simulink model "XianKongTest2022b"  (R2021a)
settings: Solver=VariableStepAuto  StartTime=0.0  StopTime=10.0  RelTol=1e-3
values from neighbouring files (symbols this model uses):
  A = [ 0 0 1 0 ... (first row only)    [fang_daolibai.m]    (also in xiankongdlb.m = [     0       0         1         0)
  B = [0;0;5.2184;-6.5125]    [fang_daolibai.m]    (also in xiankongdlb.m)
  C = [1,0,0,0;0,1,0,0]    [fang_daolibai.m]    (also in xiankongdlb.m)
  K = [  -60.6992 -316.1745  -30.0745  -33.7643]    [daolibai.m]    (also in dlfun.m = [ -60.6992 -316.1745  -30.0745  -33.7643]; fang_daolibai.m = place(A,B,P); xiankongdlb.m = place(A,B,P))
  L = place(A',C',P1)'    [fang_daolibai.m]    (also in xiankongdlb.m)
settings Model: Creator=DELL  LastModifiedBy=HanDong
settings SolverCC: AlgebraicLoopSolver=TrustRegion
settings DebuggingCC: ArithmeticOperatorsInVariantConditions=warning
settings SFSimCC: CustomCodeUndefinedFunction=UseInterfaceOnly

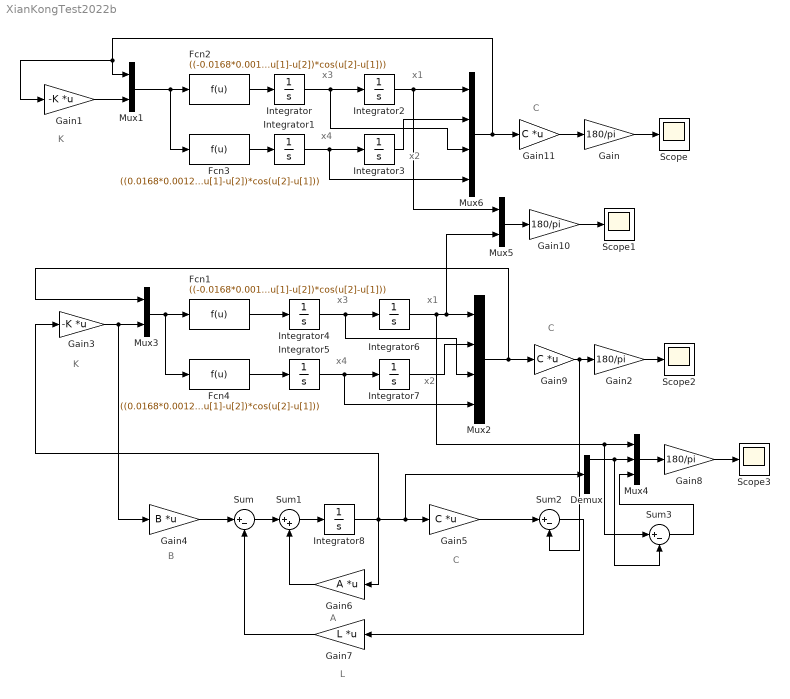
== system XianKongTest2022b ==
  note: L
  note: A
  note: B
  note: C
  note: K
  note: x4
  note: x3
  note: x2
  note: x1
  note: x1
  note: x2
  note: x3
  note: x4
  note: K
  note: C
  note: C
  Demux : Demux
  Fcn1 : Fcn  Expr=((-0.0168*0.001)*u[3]+(0.001*0.0012*cos(u[2]-u[1]))*u[4]+0.0012*0.0012*sin(u[2]-u[1])* cos(u[2]-u[1])*u[3]*u[3]-0.0012*0.001*sin(u[1]-u[2])*u[4]*u[4]+0.2979*0.001*sin(u[1])-0.0612*0.0012*sin(u[2])*cos(u[2]-u[1])+0.0236*0.001*u[5])/(0.0061*0.001-0.0012*0.0012*cos(u[1]-u[2])*cos(u[2]-u[1]))
  Fcn2 : Fcn  Expr=((-0.0168*0.001)*u[3]+(0.001*0.0012*cos(u[2]-u[1]))*u[4]+0.0012*0.0012*sin(u[2]-u[1])* cos(u[2]-u[1])*u[3]*u[3]-0.0012*0.001*sin(u[1]-u[2])*u[4]*u[4]+0.2979*0.001*sin(u[1])-0.0612*0.0012*sin(u[2])*cos(u[2]-u[1])+0.0236*0.001*u[5])/(0.0061*0.001-0.0012*0.0012*cos(u[1]-u[2])*cos(u[2]-u[1]))
  Fcn3 : Fcn  Expr=((0.0168*0.0012*cos(u[1]-u[2]))*u[3]-(0.0061*0.001)*u[4]-0.0061*0.0012*sin(u[2]-u[1])*u[3]*u[3]+0.0012*0.0012*sin(u[1]-u[2])*cos(u[1]-u[2])*u[4]*u[4]-0.2979*0.0012*sin(u[1])*cos(u[1]-u[2])+0.0061*0.0612*sin(u[2])-0.0012*cos(u[1]-u[2])*0.0236*u[5])/(0.0061*0.001-0.0012*0.0012*cos(u[1]-u[2])*cos(u[2]-u[1]))
  Fcn4 : Fcn  Expr=((0.0168*0.0012*cos(u[1]-u[2]))*u[3]-(0.0061*0.001)*u[4]-0.0061*0.0012*sin(u[2]-u[1])*u[3]*u[3]+0.0012*0.0012*sin(u[1]-u[2])*cos(u[1]-u[2])*u[4]*u[4]-0.2979*0.0012*sin(u[1])*cos(u[1]-u[2])+0.0061*0.0612*sin(u[2])-0.0012*cos(u[1]-u[2])*0.0236*u[5])/(0.0061*0.001-0.0012*0.0012*cos(u[1]-u[2])*cos(u[2]-u[1]))
  Gain{,2,8,10} (4 alike) : Gain  Gain=180/pi
  Gain1 : Gain  Gain=-K  Multiplication=Matrix(K*u)
  Gain11 : Gain  Gain=C  Multiplication=Matrix(K*u)
  Gain3 : Gain  Gain=-K  Multiplication=Matrix(K*u)
  Gain4 : Gain  Gain=B  Multiplication=Matrix(K*u)
  Gain5 : Gain  Gain=C  Multiplication=Matrix(K*u)
  Gain6 : Gain  Gain=A  Multiplication=Matrix(K*u)
  Gain7 : Gain  Gain=L  Multiplication=Matrix(K*u)
  Gain9 : Gain  Gain=C  Multiplication=Matrix(K*u)
  Integrator{,1,4..5,8} (5 alike) : Integrator
  Integrator2 : Integrator  InitialCondition=-0.1
  Integrator3 : Integrator  InitialCondition=0.05
  Integrator6 : Integrator  InitialCondition=-0.1
  Integrator7 : Integrator  InitialCondition=0.05
  Mux1 : Mux  Inputs=2
  Mux2 : Mux
  Mux3 : Mux  Inputs=2
  Mux4 : Mux  Inputs=3
  Mux5 : Mux  Inputs=2
  Mux6 : Mux
  Scope{,1..3} (4 alike) : Scope
  Sum : Sum  Inputs=|+-
  Sum1 : Sum  Inputs=|++
  Sum2 : Sum  Inputs=|+-
  Sum3 : Sum  Inputs=|+-
  wires:
  Gain/1 -> Scope/1
  Integrator2/1 -> Mux6/1, Mux5/1
  Integrator3/1 -> Mux6/2
  Integrator/1 -> Mux6/3, Integrator2/1
  Integrator1/1 -> Mux6/4, Integrator3/1
  Gain1/1 -> Mux1/2
  Mux1/1 -> Fcn3/1, Fcn2/1
  Fcn2/1 -> Integrator/1
  Fcn3/1 -> Integrator1/1
  Fcn4/1 -> Integrator5/1
  Fcn1/1 -> Integrator4/1
  Integrator5/1 -> Mux2/4, Integrator7/1
  Integrator7/1 -> Mux2/2
  Gain2/1 -> Scope2/1
  Integrator4/1 -> Mux2/3, Integrator6/1
  Mux2/1 -> Gain9/1, Mux3/1
  Gain3/1 -> Mux3/2, Gain4/1
  Mux3/1 -> Fcn4/1, Fcn1/1
  Gain4/1 -> Sum/1
  Sum/1 -> Sum1/1
  Sum1/1 -> Integrator8/1
  Integrator8/1 -> Gain3/1, Gain6/1, Demux/1, Gain5/1
  Gain5/1 -> Sum2/1
  Gain6/1 -> Sum1/2
  Gain7/1 -> Sum/2
  Sum2/1 -> Gain7/1
  Demux/1 -> Sum3/2, Mux4/2
  Sum3/1 -> Mux4/3
  Mux4/1 -> Gain8/1
  Gain8/1 -> Scope3/1
  Gain9/1 -> Sum2/2, Gain2/1
  Mux5/1 -> Gain10/1
  Gain10/1 -> Scope1/1
  Integrator6/1 -> Mux5/2, Mux2/1, Sum3/1, Mux4/1
  Gain11/1 -> Gain/1
  Mux6/1 -> Gain1/1, Mux1/1, Gain11/1
